simulink model "Exam1SysID"  (R2017a)
settings: Solver=FixedStepAuto  StartTime=0.0  StopTime=100.0  FixedStep=0.01  RelTol=1e-3  EnableMultiTasking=on
undefined symbols (not defined in the file): sigbuilder_block
libraries: simulink x3
settings Model: Creator=Sonam Tilekar  LastModifiedBy=Soutrik
settings DataIOCC: LimitDataPoints=on
settings OptimizationCC: LifeSpan=inf
settings DebuggingCC: AllowSymbolicDim=off  SFUnexpectedBacktrackingDiag=warning  SFNoUnconditionalDefaultTransitionDiag=warning  SFExecutionAtInitializationDiag=none
settings ModelReferenceCC: PropagateSignalLabelsOutOfModel=off
settings GRTTargetCC: TargetLangStandard=C89/C90 (ANSI)
settings ConfigComp: CovMetricSettings=dw  CovHtmlReporting=on  CovSaveCumulativeToWorkspaceVar=on  CovSaveSingleToWorkspaceVar=on  CovExternalEMLEnable=off

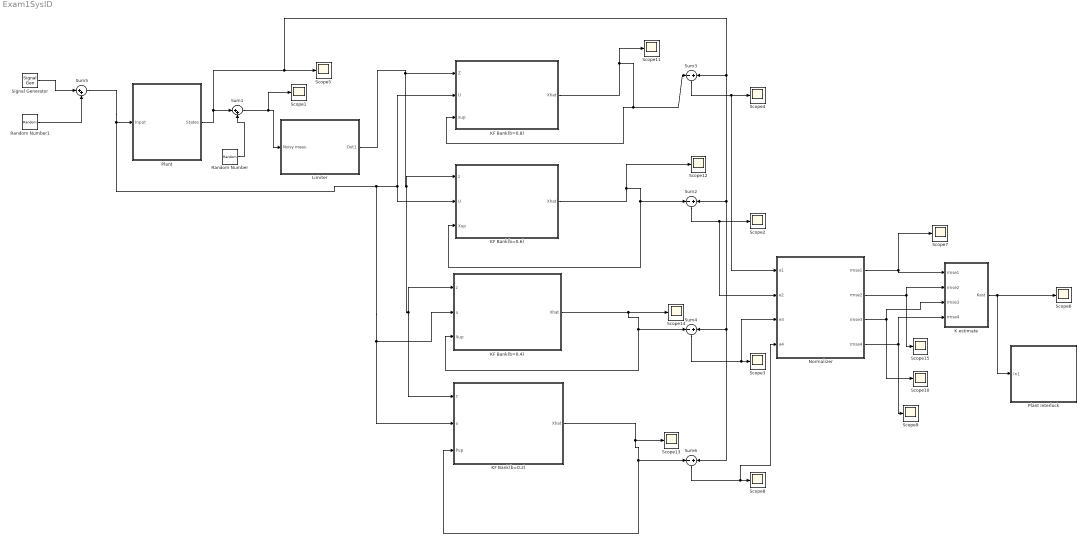
== system Exam1SysID ==
  K estimate : MATLAB Function  TreatAsAtomicUnit=on
  KF Bank(b=0.2) : Subsystem
  KF Bank(b=0.4) : Subsystem
  KF Bank(b=0.6) : Subsystem
  KF Bank(b=0.8) : Subsystem
  Limiter : Subsystem
  Normalizer : MATLAB Function  TreatAsAtomicUnit=on
  Plant : Subsystem
  Plant Interlock : Subsystem
  Random Number : RandomNumber  Variance=0.001  Seed=47  SampleTime=0.01
  Random Number1 : RandomNumber  Variance=0.001  Seed=67  SampleTime=0.01
  Scope{1..15} (15 alike) : Scope
  Signal Generator : SignalGenerator  WaveForm=square  Frequency=0.1
  Sum1 : Sum  Inputs=|++
  Sum{2..4,6} (4 alike) : Sum  Inputs=-+
  Sum5 : Sum  Inputs=|++
  wires:
  Random Number/1 -> Sum1/2
  Sum4/1 -> Normalizer/3(e3), Scope3/1
  Sum3/1 -> Normalizer/1(e1), Scope4/1
  Sum2/1 -> Normalizer/2(e2), Scope2/1
  Normalizer/1(rmse1) -> Scope7/1, K estimate/1(rmse1)
  Normalizer/2(rmse2) -> K estimate/2(rmse2), Scope15/1
  Normalizer/3(rmse3) -> K estimate/3(rmse3), Scope10/1
  K estimate/1(Kest) -> Plant Interlock/1(In1), Scope6/1
  Sum6/1 -> Normalizer/4(e4), Scope8/1
  Normalizer/4(rmse4) -> K estimate/4(rmse4), Scope9/1
  KF Bank(b=0.8)/1(Xhat) -> Scope11/1, KF Bank(b=0.8)/3(xup), Sum3/1
  Plant/1(States) -> Scope5/1, Sum3/2, Sum6/2, Sum4/2, Sum2/2, Sum1/1
  Signal Generator/1 -> Sum5/1
  Random Number1/1 -> Sum5/2
  Sum5/1 -> KF Bank(b=0.2)/2(u), KF Bank(b=0.4)/2(u), KF Bank(b=0.6)/2(U), KF Bank(b=0.8)/2(U), Plant/1(Input)
  KF Bank(b=0.6)/1(Xhat) -> Scope12/1, KF Bank(b=0.6)/3(Xup), Sum2/1
  KF Bank(b=0.4)/1(Xhat) -> KF Bank(b=0.4)/3(Xup), Sum4/1, Scope14/1
  KF Bank(b=0.2)/1(Xhat) -> KF Bank(b=0.2)/3(Pup), Sum6/1, Scope13/1
  Sum1/1 -> Scope1/1, Limiter/1(Noisy meas.)
  Limiter/1(Out1) -> KF Bank(b=0.2)/1(z), KF Bank(b=0.4)/1(z), KF Bank(b=0.6)/1(z), KF Bank(b=0.8)/1(Z)

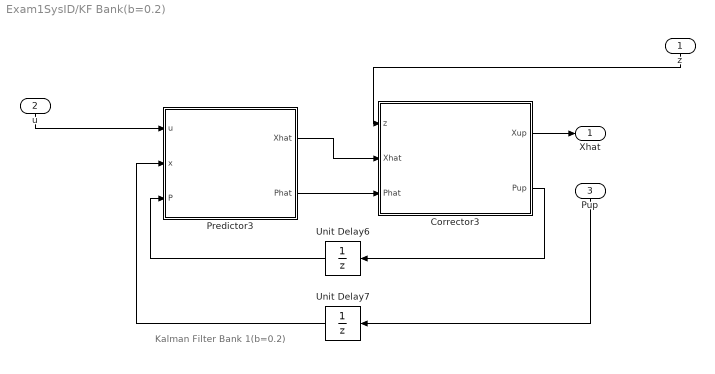
== system Exam1SysID/KF Bank(b=0.2) ==
  note: Kalman Filter Bank 1(b=0.2)
  z : Inport
  u : Inport  Port=2
  Pup : Inport  Port=3
  Corrector3 : MATLAB Function  TreatAsAtomicUnit=on
  Predictor3 : MATLAB Function  TreatAsAtomicUnit=on
  Unit Delay6 : UnitDelay  InitialCondition=eye(2)  SampleTime=0.01
  Unit Delay7 : UnitDelay  InitialCondition=[0;0]  SampleTime=0.01
  Xhat : Outport
  wires:
  Corrector3/2(Pup) -> Unit Delay6/1
  Predictor3/2(Phat) -> Corrector3/3(Phat)
  Unit Delay7/1 -> Predictor3/2(x)
  Corrector3/1(Xup) -> Xhat/1
  Unit Delay6/1 -> Predictor3/3(P)
  Predictor3/1(Xhat) -> Corrector3/2(Xhat)
  u/1 -> Predictor3/1(u)
  Pup/1 -> Unit Delay7/1
  z/1 -> Corrector3/1(z)

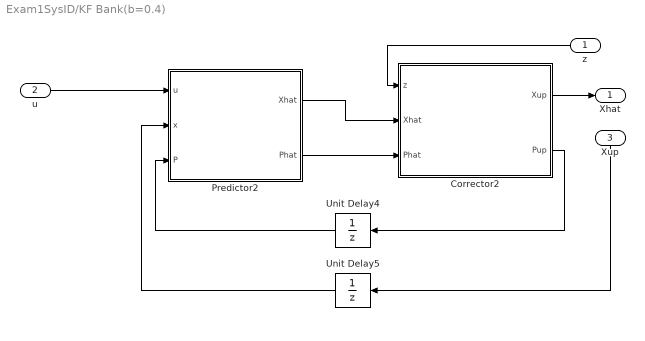
== system Exam1SysID/KF Bank(b=0.4) ==
  z : Inport
  u : Inport  Port=2
  Xup : Inport  Port=3
  Corrector2 : MATLAB Function  TreatAsAtomicUnit=on
  Predictor2 : MATLAB Function  TreatAsAtomicUnit=on
  Unit Delay4 : UnitDelay  InitialCondition=eye(2)  SampleTime=0.01
  Unit Delay5 : UnitDelay  InitialCondition=[0;0]  SampleTime=0.01
  Xhat : Outport
  wires:
  Xup/1 -> Unit Delay5/1
  z/1 -> Corrector2/1(z)
  u/1 -> Predictor2/1(u)
  Predictor2/2(Phat) -> Corrector2/3(Phat)
  Predictor2/1(Xhat) -> Corrector2/2(Xhat)
  Unit Delay4/1 -> Predictor2/3(P)
  Unit Delay5/1 -> Predictor2/2(x)
  Corrector2/2(Pup) -> Unit Delay4/1
  Corrector2/1(Xup) -> Xhat/1

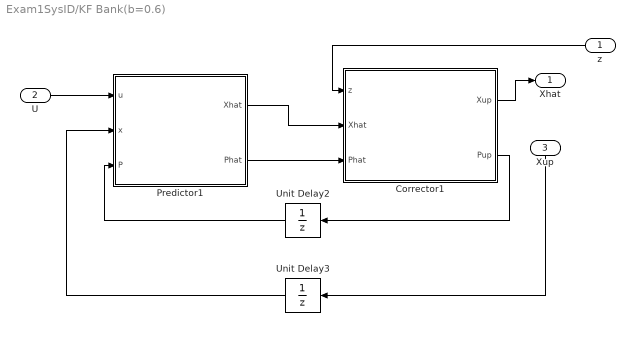
== system Exam1SysID/KF Bank(b=0.6) ==
  z : Inport
  U : Inport  Port=2
  Xup : Inport  Port=3
  Corrector1 : MATLAB Function  TreatAsAtomicUnit=on
  Predictor1 : MATLAB Function  TreatAsAtomicUnit=on
  Unit Delay2 : UnitDelay  InitialCondition=eye(2)  SampleTime=0.01
  Unit Delay3 : UnitDelay  InitialCondition=[0;0]  SampleTime=0.01
  Xhat : Outport
  wires:
  Xup/1 -> Unit Delay3/1
  z/1 -> Corrector1/1(z)
  U/1 -> Predictor1/1(u)
  Corrector1/2(Pup) -> Unit Delay2/1
  Predictor1/1(Xhat) -> Corrector1/2(Xhat)
  Corrector1/1(Xup) -> Xhat/1
  Unit Delay3/1 -> Predictor1/2(x)
  Predictor1/2(Phat) -> Corrector1/3(Phat)
  Unit Delay2/1 -> Predictor1/3(P)

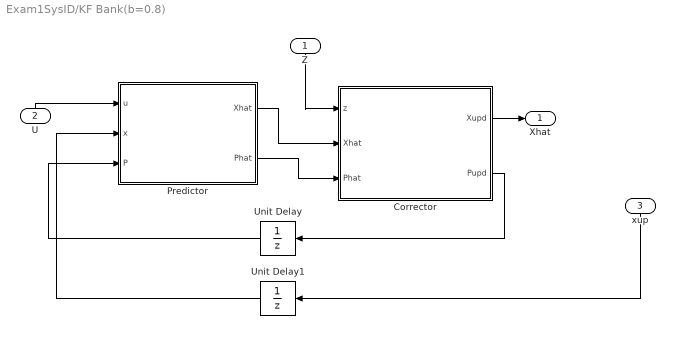
== system Exam1SysID/KF Bank(b=0.8) ==
  Z : Inport
  U : Inport  Port=2
  xup : Inport  Port=3
  Corrector : MATLAB Function  TreatAsAtomicUnit=on
  Predictor : MATLAB Function  TreatAsAtomicUnit=on
  Unit Delay : UnitDelay  InitialCondition=eye(2)  SampleTime=0.01
  Unit Delay1 : UnitDelay  InitialCondition=[0;0]  SampleTime=0.01
  Xhat : Outport
  wires:
  Predictor/2(Phat) -> Corrector/3(Phat)
  Predictor/1(Xhat) -> Corrector/2(Xhat)
  Unit Delay/1 -> Predictor/3(P)
  Unit Delay1/1 -> Predictor/2(x)
  Corrector/2(Pupd) -> Unit Delay/1
  Corrector/1(Xupd) -> Xhat/1
  xup/1 -> Unit Delay1/1
  Z/1 -> Corrector/1(z)
  U/1 -> Predictor/1(u)

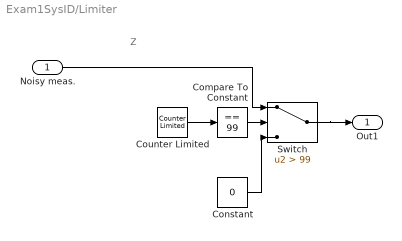
== system Exam1SysID/Limiter ==
  note: Z
  Noisy meas. : Inport
  Compare To Constant : simulink/Logic and Bit Operations/Compare To Constant  relop===  const=99  OutDataTypeStr=boolean
  Constant : Constant  Value=0
  Counter Limited : simulink/Sources/Counter Limited  uplimit=99  tsamp=0.01
  Switch : Switch  Criteria=u2 > Threshold  Threshold=99
  Out1 : Outport
  wires:
  Noisy meas./1 -> Switch/1
  Compare To Constant/1 -> Switch/2
  Constant/1 -> Switch/3
  Switch/1 -> Out1/1
  Counter Limited/1 -> Compare To Constant/1

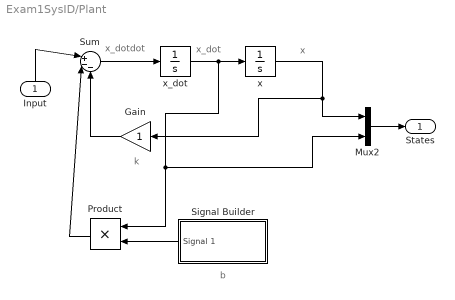
== system Exam1SysID/Plant ==
  note: x
  note: k
  note: x_dot
  note: x_dotdot
  note: b
  Input : Inport
  Gain : Gain
  Mux2 : Mux  Inputs=2
  Product : Product
  Signal Builder : Subsystem  Tag=STV Subsys  LoadFcn=sigbuilder_block('load');  StartFcn=sigbuilder_block('start');  StopFcn=sigbuilder_block('stop');  ClipboardFcn=sigbuilder_block('clipboard');  mask(Sigbuilder block){tuvar=[0:10]}
      mask help: Simulink:masks:SigbuilderBlock_MD
      mask init:
      | if ~strcmp(get_param(bdroot(gcbh),'SimulationStatus'),'stopped') tuvar = sigbuilder_block('maskInit'); end
      settings: CopyFcn=sigbuilder_block('copy');  DeleteFcn=sigbuilder_block('delete');  ModelCloseFcn=sigbuilder_block('modelClose');  PreSaveFcn=sigbuilder_block('preSave');  PauseFcn=sigbuilder_block('pause');  ContinueFcn=sigbuilder_block('continue');  NameChangeFcn=sigbuilder_block('namechange');  OpenFcn=sigbuilder_block('open',[0 30 1026 601.5 ]);  CloseFcn=sigbuilder_block('close');
      mask Display: plot(0, 0, 100, 100,[2, 2, 32, 32, 2], [68, 8, 8, 68, 68],[32, 2], [38, 38], [32, 19, 2],[53, 60, 44], [32, 17, 17, 2],[16, 16, 31, 31]);txt = getActiveGroup(gcbh);text(2, 100, txt,'verticalAlignment', 'top');
  Sum : Sum  Inputs=|+--
  x : Integrator
  x_dot : Integrator
  States : Outport
  wires:
  Signal Builder/1(Signal 1) -> Product/2
  x/1 -> Gain/1, Mux2/1
  x_dot/1 -> Mux2/2, Product/1, x/1
  Sum/1 -> x_dot/1
  Product/1 -> Sum/2
  Gain/1 -> Sum/3
  Mux2/1 -> States/1
  Input/1 -> Sum/1

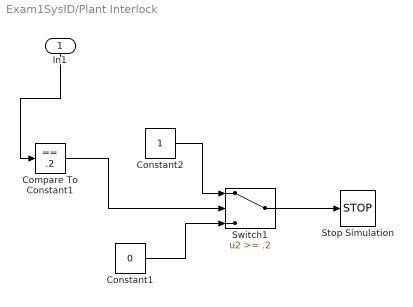
== system Exam1SysID/Plant Interlock ==
  In1 : Inport
  Compare To Constant1 : simulink/Logic and Bit Operations/Compare To Constant  relop===  const=.2  OutDataTypeStr=boolean
  Constant1 : Constant  Value=0
  Constant2 : Constant
  Stop Simulation : Stop
  Switch1 : Switch  Threshold=.2
  wires:
  Constant1/1 -> Switch1/3
  Switch1/1 -> Stop Simulation/1
  Constant2/1 -> Switch1/1
  In1/1 -> Compare To Constant1/1
  Compare To Constant1/1 -> Switch1/2

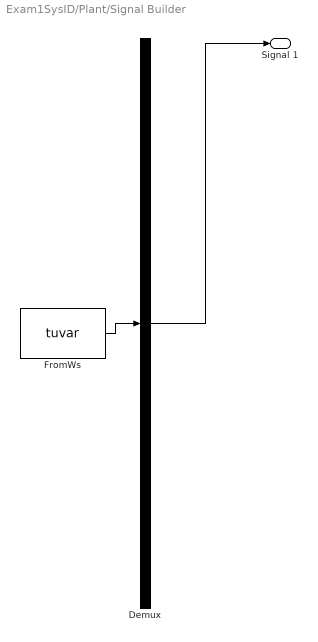
== system Exam1SysID/Plant/Signal Builder ==
  Demux : Demux  Tag=STV Demux  Outputs=1
  FromWs : FromWorkspace  Tag=STV FromWs  VariableName=tuvar  SampleTime=0
      SigBuilderData=|
      | common.afterFinalStr = 'Extrapolate'
      | common.sampleTime = 0
      | dataSet.timeRange = [0 100]
      | dataSet.name = 'Group 1'
      | sbobj.Groups.Name = 'Group 1'
      | sbobj.Groups.Signals.Name = 'Signal 1'
      | sbobj.Groups.Signals.XData = [0 24 24 55 55 76 76 100]
      | sbobj.Groups.Signals.YData = [0.8 0.8 0.6 0.6 0.4 0.4 0.2 0.2]
      | sbobj.Groups.TimeRange = [0 100]
  Signal 1 : Outport  Tag=STV Outport
  wires:
  Demux/1 -> Signal 1/1
  FromWs/1 -> Demux/1

== matlab function Exam1SysID/KF Bank(b=0.8)/Corrector ==
  data: z input; Xupd output; Xhat input; Phat input; Pupd output
function [Xupd,Pupd] = corrector(z,Xhat,Phat)
h=eye(2);
r=eye(2);
if z(1) == 0 && z(2) == 0
    Xupd = Xhat;
    Pupd = Phat;
else
    rd= 1 /0.01 * r;
    K=Phat*h'*inv(h*Phat*h'+rd);
    Pupd=(eye(2)-K*h)*Phat*(eye(2)-K*h)'+K*rd*K';
    Xupd=Xhat+K*(z-h*Xhat);
end
end

== matlab function Exam1SysID/KF Bank(b=0.8)/Predictor ==
  data: u input; Xhat output; Phat output; x input; P input
function [Xhat,Phat] = Predictor(u,x,P)
Q=10*eye(2);b =[0; 1];
a=[0 1;-1 -.8]; %[0 1;-k -b]
ad=expm(a*0.01);
bd=inv(a)*(ad-eye(2))*b;
f=[-a Q;
   zeros(2,2) a'];
g=expm(f*0.01);
Qd=g(3:4,3:4)'*g(1:2,3:4);
Xhat=ad*x+bd*u;                 %State prediction
Phat=ad*P+ad'*Qd;               %Covariance prediction
end

== matlab function Exam1SysID/KF Bank(b=0.6)/Corrector1 ==
  data: z input; Xup output; Xhat input; Phat input; Pup output
function [Xup,Pup] = corrector(z,Xhat,Phat)
h=eye(2);
r=eye(2);
if z(1) == 0 && z(2) == 0
    Xup = Xhat;
    Pup = Phat;
else
    rd= 1 /0.01 * r;
    k=Phat*h'*inv(h*Phat*h'+rd);
    Pup=(eye(2)-k*h)*Phat*(eye(2)-k*h)'+k*rd*k';
    Xup=Xhat+k*(z-h*Xhat);
end
end

== matlab function Exam1SysID/KF Bank(b=0.6)/Predictor1 ==
  data: u input; Xhat output; Phat output; x input; P input
function [Xhat,Phat] = Predictor(u,x,P)
a=[0 1;-1 -0.6]; %[0 1;-b -k]
Q=6*eye(2);b =[0; 1];
ad=expm(a*0.01);
bd=inv(a)*(ad-eye(2))*b;
f=[-a Q;
   zeros(2,2) a'];
g=expm(f*0.01);
Qd=g(3:4,3:4)'*g(1:2,3:4);
Xhat=ad*x+bd*u;                 %State prediction
Phat=ad*P+ad'*Qd;               %Covariance prediction
end

== matlab function Exam1SysID/KF Bank(b=0.4)/Corrector2 ==
  data: z input; Xhat input; Phat input; Xup output; Pup output
function [Xup,Pup] = corrector(z,Xhat,Phat)
h=eye(2);
r=eye(2);
if z(1) == 0 && z(2) == 0
    Xup = Xhat;
    Pup = Phat;
else
    rd= 1 /0.01 * r;
    k=Phat*h'*inv(h*Phat*h'+rd);
    Pup=(eye(2)-k*h)*Phat*(eye(2)-k*h)'+k*rd*k';
    Xup=Xhat+k*(z-h*Xhat);
end
end

== matlab function Exam1SysID/KF Bank(b=0.4)/Predictor2 ==
  data: u input; Xhat output; Phat output; x input; P input
function [Xhat,Phat] = Predictor(u,x,P)
a=[0 1;-1 -.4]; 
Q=10*eye(2);b =[0; 1];
ad=expm(a*0.01);
bd=inv(a)*(ad-eye(2))*b;
f=[-a Q;
   zeros(2,2) a'];
g=expm(f*0.01);
Qd=g(3:4,3:4)'*g(1:2,3:4);
Xhat=ad*x+bd*u;                 %State prediction
Phat=ad*P+ad'*Qd;               %Covariance prediction
end

== matlab function Exam1SysID/KF Bank(b=0.2)/Corrector3 ==
  data: z input; Xup output; Xhat input; Phat input; Pup output
function [Xup,Pup] = corrector(z,Xhat,Phat)
h=eye(2);
r=eye(2);
if z(1) == 0 && z(2) == 0
    Xup = Xhat;
    Pup = Phat;
else
    rd= 1 /0.01 * r;
    K=Phat*h'*inv(h*Phat*h'+rd);
    Pup=(eye(2)-K*h)*Phat*(eye(2)-K*h)'+K*rd*K';
    Xup=Xhat+K*(z-h*Xhat);
end
end

== matlab function Exam1SysID/KF Bank(b=0.2)/Predictor3 ==
  data: u input; Xhat output; Phat output; x input; P input
function [Xhat,Phat] = Predictor(u,x,P)
a=[0 1;-1 -0.2]; 
Q=10*eye(2);b =[0; 1];
ad=expm(a*0.01);
Bd=inv(a)*(ad-eye(2))*b;
f=[-a Q;
   zeros(2,2) a'];
g=expm(f*0.01);
Qd=g(3:4,3:4)'*g(1:2,3:4);
Xhat=ad*x+Bd*u;            %State prediction
Phat=ad*P+ad'*Qd;          %Covariance prediction
end

== matlab function Exam1SysID/Normalizer ==
  data: e1 input; rmse1 output; e2 input; e3 input; e4 input; rmse2 output; rmse3 output; rmse4 output
function [rmse1,rmse2,rmse3,rmse4] = rmse(e1,e2,e3,e4)

rmse1=sqrt(e1(1)^2+e1(2)^2);
rmse2=sqrt(e2(1)^2+e2(2)^2);
rmse3=sqrt(e3(1)^2+e3(2)^2);
rmse4=sqrt(e4(1)^2+e4(2)^2);
end

== matlab function Exam1SysID/K estimate ==
  data: rmse1 input; Kest output; rmse2 input; rmse3 input; rmse4 input
function Kest = fcn(rmse1,rmse2,rmse3,rmse4)

[j,k]=min([rmse1,rmse2,rmse3,rmse4]);
Kest=.8;
switch k
    case 1
        Kest=.8;
    case 2
        Kest=0.6;
    case 3
        Kest=0.4;
    case 4
        Kest=0.2;
end
end
